simulink model "rohr_1"  (Simulink 4.00)
settings: Solver=ode23s  StartTime=0.0  StopTime=200  MaxStep=0.1  RelTol=10e-3
libraries: simulink3 x1
settings Model: LastModifiedBy=Administrator  Refine=5  BlockReductionOpt=off

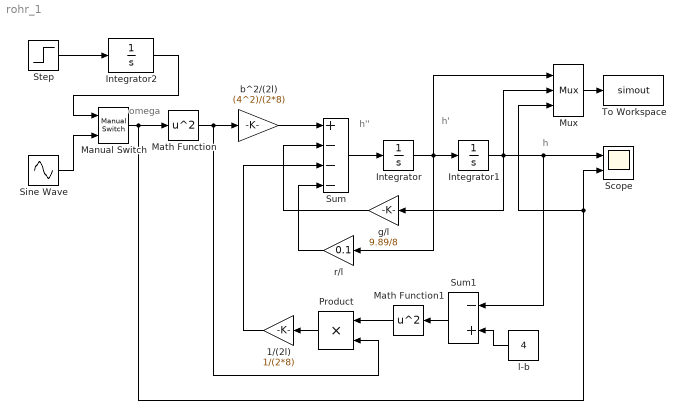
== system rohr_1 ==
  note: h''
  note: h'
  note: h
  note: omega
  1/(2l) : Gain  Orientation=left  Gain=1/(2*8)  Multiplication=Element-wise(K.*u)  SaturateOnIntegerOverflow=on
  Integrator : Integrator  ExternalReset=none  InitialConditionSource=internal  InitialCondition=0  LimitOutput=off  UpperSaturationLimit=inf  LowerSaturationLimit=-inf  ShowSaturationPort=off  ShowStatePort=off  AbsoluteTolerance=auto
  Integrator1 : Integrator  ExternalReset=none  InitialConditionSource=internal  InitialCondition=1  LimitOutput=off  UpperSaturationLimit=inf  LowerSaturationLimit=-inf  ShowSaturationPort=off  ShowStatePort=off  AbsoluteTolerance=auto
  Integrator2 : Integrator  ExternalReset=none  InitialConditionSource=internal  InitialCondition=0  LimitOutput=on  UpperSaturationLimit=1.5  LowerSaturationLimit=-inf  ShowSaturationPort=off  ShowStatePort=off  AbsoluteTolerance=auto
  Manual Switch : simulink3/Nonlinear/Manual Switch  sw=1  action=0
  Math Function : Math  Operator=square  OutputSignalType=auto
  Math Function1 : Math  Orientation=left  Operator=square  OutputSignalType=auto
  Mux : Mux  Inputs=3
      settings: DisplayOption=none
  Product : Product  Orientation=left  Inputs=2  Multiplication=Element-wise(.*)  SaturateOnIntegerOverflow=on
  Scope : Scope  NumInputPorts=2
      settings: TimeRange=auto  YMin=-1~-0.5  YMax=1~0.5  SaveToWorkspace=off  SaveName=ScopeData  MaxDataPoints=5000
  Sine Wave : Sin  Amplitude=0.5  Frequency=0.99  Phase=0  SampleTime=0
  Step : Step  Time=0  Before=0  After=0.01  SampleTime=0
  Sum : Sum  Inputs=+---  SaturateOnIntegerOverflow=on
  Sum1 : Sum  Orientation=left  Inputs=-+  SaturateOnIntegerOverflow=on
  To Workspace : ToWorkspace  VariableName=simout  SampleTime=-1  SaveFormat=Structure
  b^2/(2l) : Gain  Gain=(4^2)/(2*8)  Multiplication=Element-wise(K.*u)  SaturateOnIntegerOverflow=on
  g/l : Gain  Orientation=left  Gain=9.89/8  Multiplication=Element-wise(K.*u)  SaturateOnIntegerOverflow=on
  l-b : Constant  Orientation=left  Value=4
  r/l : Gain  Orientation=left  Gain=0.1  Multiplication=Element-wise(K.*u)  SaturateOnIntegerOverflow=on
  wires:
  Math Function/1 -> b^2/(2l)/1, Product/2
  b^2/(2l)/1 -> Sum/1
  Sum/1 -> Integrator/1
  Integrator/1 -> Integrator1/1, r/l/1, Mux/1
  Integrator1/1 -> Sum1/1, Scope/1, g/l/1, Mux/2
  l-b/1 -> Sum1/2
  Sum1/1 -> Math Function1/1
  Math Function1/1 -> Product/1
  Product/1 -> 1/(2l)/1
  1/(2l)/1 -> Sum/3
  Manual Switch/1 -> Math Function/1, Scope/2, Mux/3
  g/l/1 -> Sum/2
  r/l/1 -> Sum/4
  Sine Wave/1 -> Manual Switch/2
  Step/1 -> Integrator2/1
  Integrator2/1 -> Manual Switch/1
  Mux/1 -> To Workspace/1
